simulink model "current_contour"  (R2023a)
settings: Solver=VariableStepAuto  StartTime=0.0  StopTime=0.2  MaxStep=1e-4  RelTol=1e-3
undefined symbols (not defined in the file or in its folder): i, J, k_curr, k_pow, k_spd, ki_curr, km, kp_curr, kw, R, T_e, T_pow
settings Model: Creator=k.balkunov  LastModifiedBy=k.balkunov

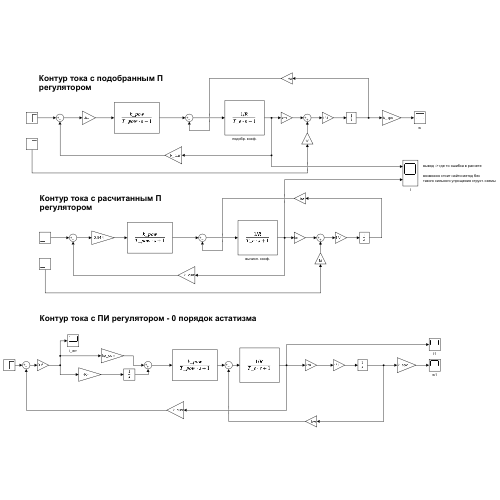
[thumbnail: Simulink's stored preview of the top-level diagram]
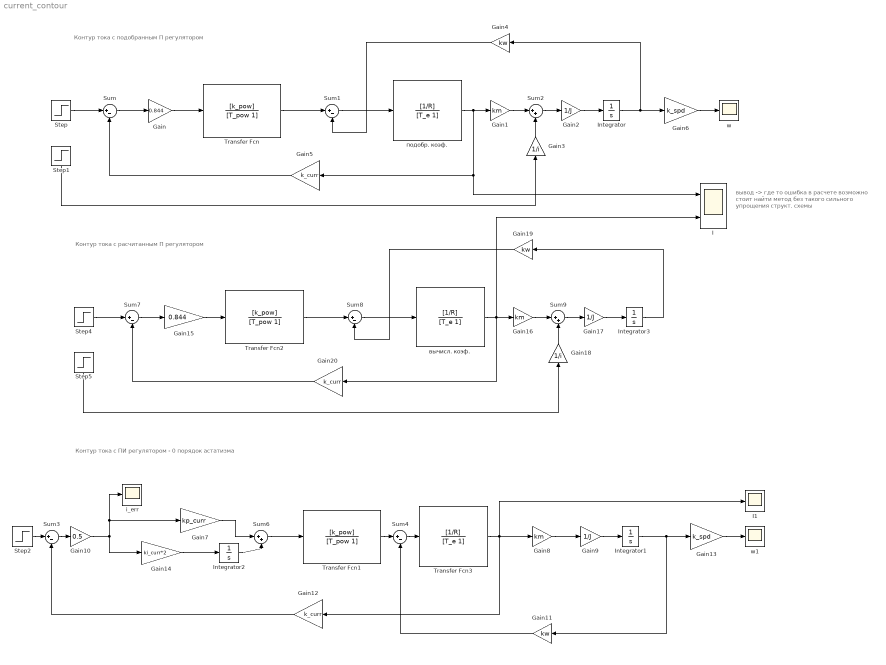
== system current_contour ==
  note: вывод -> где то ошибка в расчете
      |
      | возможно стоит найти метод без
      | такого сильного упрощения структ. схемы
  note: Контур тока с подобранным П регулятором
  note: Контур тока с ПИ регулятором - 0 порядок астатизма
  note: Контур тока с расчитанным П регулятором
  Gain : Gain  Gain=0.844
  Gain1 : Gain  Gain=km
  Gain10 : Gain  Gain=0.5
  Gain11 : Gain  Gain=kw
  Gain12 : Gain  Gain=k_curr
  Gain13 : Gain  Gain=k_spd
  Gain14 : Gain  Gain=ki_curr*2
  Gain15 : Gain  Gain=0.844
  Gain16 : Gain  Gain=km
  Gain17 : Gain  Gain=1/J
  Gain18 : Gain  Gain=1/i
  Gain19 : Gain  Gain=kw
  Gain2 : Gain  Gain=1/J
  Gain20 : Gain  Gain=k_curr
  Gain3 : Gain  Gain=1/i
  Gain4 : Gain  Gain=kw
  Gain5 : Gain  Gain=k_curr
  Gain6 : Gain  Gain=k_spd
  Gain7 : Gain  Gain=kp_curr
  Gain8 : Gain  Gain=km
  Gain9 : Gain  Gain=1/J
  I : Scope  NumInputPorts=2
  I1 : Scope
  Integrator{,1..3} (4 alike) : Integrator
  Step : Step  Time=0  SampleTime=0
  Step1 : Step  Time=5  SampleTime=0
  Step2 : Step  Time=0  SampleTime=0
  Step4 : Step  Time=0  SampleTime=0
  Step5 : Step  Time=5  SampleTime=0
  Sum{,1,3..4,7..8} (6 alike) : Sum  Inputs=|+-
  Sum2 : Sum  Inputs=|++
  Sum6 : Sum  Inputs=|++
  Sum9 : Sum  Inputs=|++
  Transfer Fcn : TransferFcn  Numerator=[k_pow]  Denominator=[T_pow 1]
  Transfer Fcn1 : TransferFcn  Numerator=[k_pow]  Denominator=[T_pow 1]
  Transfer Fcn2 : TransferFcn  Numerator=[k_pow]  Denominator=[T_pow 1]
  Transfer Fcn3 : TransferFcn  Numerator=[1/R]  Denominator=[T_e 1]
  i_err : Scope
  w : Scope
  w1 : Scope
  вычисл. коэф. : TransferFcn  Numerator=[1/R]  Denominator=[T_e 1]
  подобр. коэф. : TransferFcn  Numerator=[1/R]  Denominator=[T_e 1]
  wires:
  Gain/1 -> Transfer Fcn/1
  Transfer Fcn/1 -> Sum1/1
  Sum1/1 -> подобр. коэф./1
  Sum/1 -> Gain/1
  подобр. коэф./1 -> I/1, Gain5/1, Gain1/1
  Step/1 -> Sum/1
  Gain2/1 -> Integrator/1
  Sum2/1 -> Gain2/1
  Gain1/1 -> Sum2/1
  Step1/1 -> Gain3/1
  Gain3/1 -> Sum2/2
  Integrator/1 -> Gain4/1, Gain6/1
  Gain4/1 -> Sum1/2
  Gain5/1 -> Sum/2
  Gain6/1 -> w/1
  Gain11/1 -> Sum4/2
  Gain13/1 -> w1/1
  Transfer Fcn3/1 -> Gain8/1, Gain12/1, I1/1
  Gain12/1 -> Sum3/2
  Sum4/1 -> Transfer Fcn3/1
  Gain9/1 -> Integrator1/1
  Integrator1/1 -> Gain11/1, Gain13/1
  Gain8/1 -> Gain9/1
  Step2/1 -> Sum3/1
  Sum8/1 -> вычисл. коэф./1
  Sum7/1 -> Gain15/1
  Gain17/1 -> Integrator3/1
  Gain19/1 -> Sum8/2
  Transfer Fcn2/1 -> Sum8/1
  Sum9/1 -> Gain17/1
  Gain18/1 -> Sum9/2
  Gain20/1 -> Sum7/2
  Gain16/1 -> Sum9/1
  Integrator3/1 -> Gain19/1
  Step4/1 -> Sum7/1
  вычисл. коэф./1 -> Gain20/1, I/2, Gain16/1
  Gain15/1 -> Transfer Fcn2/1
  Step5/1 -> Gain18/1
  Transfer Fcn1/1 -> Sum4/1
  Gain14/1 -> Integrator2/1
  Gain7/1 -> Sum6/1
  Integrator2/1 -> Sum6/2
  Sum6/1 -> Transfer Fcn1/1
  Sum3/1 -> Gain10/1
  Gain10/1 -> i_err/1, Gain7/1, Gain14/1
